simulink model "PowerSplitDriveUnit_harness_model"  (R2022a)
settings: Solver=daessc  StartTime=0.0  StopTime=t_end  RelTol=1e-3  AbsTol=1e-3
PreLoadFcn:
  | PowerSplitDriveUnit_harness_setup
libraries: fl_lib x7, nesl_utility x6, sdl_lib x1
settings Model: Creator=isaacito  LastModifiedBy=isaacito
settings SolverCC: AutoScaleAbsTol=off  AlgebraicLoopSolver=TrustRegion
settings DataIOCC: DSMLogging=off  InspectSignalLogs=on
settings DebuggingCC: UnconnectedInputMsg=warning  UnconnectedOutputMsg=warning  UnconnectedLineMsg=warning  SFMachineParentedDataDiag=warning
settings RTWCC: DLArmComputeVersion=19.05
settings SimscapeCC: SimscapeLogType=all  SimscapeLogSimulationStatistics=on  SimscapeLogLimitData=off

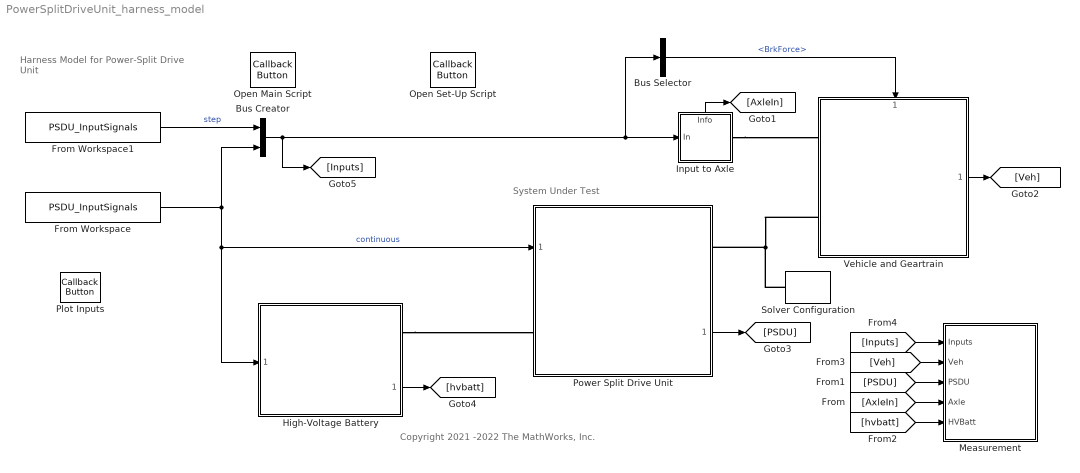
== system PowerSplitDriveUnit_harness_model ==
  note: System Under Test
  note: Copyright 2021 -2022 The MathWorks, Inc.
  note: Harness Model for
      | Power-Split Drive Unit
  Bus Creator : BusCreator  Inputs=2
  Bus Selector : BusSelector  OutputSignals=continuous.BrkForce
  From Workspace : FromWorkspace  VariableName=PSDU_InputSignals  OutDataTypeStr=Bus: PSDU_InputBus  OutputAfterFinalValue=Holding final value
      settings: AttributesFormatString=|
      | %<OutDataTypeStr>
      | Interpolate: %<Interpolate>
  From Workspace1 : FromWorkspace  VariableName=PSDU_InputSignals  OutDataTypeStr=Bus: PSDU_InputBus  Interpolate=off  OutputAfterFinalValue=Holding final value
      settings: AttributesFormatString=|
      | %<OutDataTypeStr>
      | Interpolate: %<Interpolate>
  High-Voltage Battery : Subsystem  ReferencedSubsystem=BatteryForTest2_refsub
      settings: PortSchema="{\"entries\":[{\"content\":{\"sides\":[{\"content\":{\"connectorIds\":[\"In1\"]},\"type\":\"ConnectorPlacement.EquallySpacedRectSide\",\"uuid\":\"6ec42dc2-af13-403d-bb44-bbfe17049ebb\"},{\"content\":{\"connectorIds\":[\"RConn1\",\"Out1\"],\"side\":\"RIGHT\"},\"type\":\"ConnectorPlacement.EquallySpacedRectSide\",\"uuid\":\"18b43a22-b216-415c-b9ff-5dd426481655\"},{\"content\":{\"connectorIds\":[],\"side\":\"TOP\"},\"type\":\"ConnectorPlacement.EquallySpacedRectSide\",\"uuid\":\"9ddf6635-2c27-427a-8c83-df626a0e9ed3\"},{\"content\":{\"connectorIds\":[],\"side\":\"HIDDEN\"},\"type\":\"ConnectorPlacement.EquallySpacedRectSide\",\"uuid\":\"332981be-c8a8-46f3-86be-153015cc7779\"}]},\"type\":\"ConnectorPlacement.EquallySpacedConnector\",\"uuid\":\"0a64d723-305c-452f-a915-e14881ea19f7\"}],\"packageUris\":[\"http://schema.mathworks.com/mf0/Connector/R2020b\"],\"version\":\"1.0\"}"
  Input to Axle : Subsystem
      settings: PortSchema="{\"entries\":[{\"content\":{\"sides\":[{\"content\":{\"connectorIds\":[\"In1\"]},\"type\":\"ConnectorPlacement.EquallySpacedRectSide\",\"uuid\":\"17ecda4f-ad99-4587-a38d-a324d7486455\"},{\"content\":{\"connectorIds\":[\"RConn1\"],\"side\":\"RIGHT\"},\"type\":\"ConnectorPlacement.EquallySpacedRectSide\",\"uuid\":\"02def29b-e53d-45c2-af98-8005350a1631\"},{\"content\":{\"connectorIds\":[\"Out1\"],\"side\":\"TOP\"},\"type\":\"ConnectorPlacement.EquallySpacedRectSide\",\"uuid\":\"2d06855e-5bd1-4c4c-a72f-3146430204d1\"}]},\"type\":\"ConnectorPlacement.EquallySpacedConnector\",\"uuid\":\"a8d07ca5-35bb-4517-a87a-8359777d2cb9\"}],\"packageUris\":[\"http://schema.mathworks.com/mf0/Connector/R2020b\"],\"version\":\"1.0\"}"
  Measurement : Subsystem
  Open Main Script : CallbackButton  ButtonText=Open
      settings: ClickFcn=edit PowerSplitDriveUnit_main_script
  Open Set-Up Script : CallbackButton  ButtonText=Open
      settings: ClickFcn=edit PowerSplitDriveUnit_harness_setup.m
  Plot Inputs : CallbackButton  ButtonText=Plot
      settings: ClickFcn="PowerSplitDriveUnit_plot_inputs(\"PSDU_InputSignals\")"
  Power Split Drive Unit : Subsystem  ReferencedSubsystem=PowerSplitDriveUnitBasic_refsub
      settings: PortSchema="{\"entries\":[{\"content\":{\"sides\":[{\"content\":{\"connectorIds\":[\"In1\",\"LConn1\"]},\"type\":\"ConnectorPlacement.EquallySpacedRectSide\",\"uuid\":\"ac3719a4-f5ca-49c1-b88d-60ddfcbc9c3c\"},{\"content\":{\"connectorIds\":[\"RConn1\",\"Out1\"],\"side\":\"RIGHT\"},\"type\":\"ConnectorPlacement.EquallySpacedRectSide\",\"uuid\":\"02c1cdca-c4bc-4e36-8da7-b9fd13165580\"},{\"content\":{\"connectorIds\":[],\"side\":\"TOP\"},\"type\":\"ConnectorPlacement.EquallySpacedRectSide\",\"uuid\":\"9a293679-982e-42e0-b445-a53b2f9deeb2\"},{\"content\":{\"connectorIds\":[],\"side\":\"HIDDEN\"},\"type\":\"ConnectorPlacement.EquallySpacedRectSide\",\"uuid\":\"92624000-5028-4c46-b75d-fdf82f03c691\"}]},\"type\":\"ConnectorPlacement.EquallySpacedConnector\",\"uuid\":\"49b414d9-6436-4fd3-904c-291d56adec0c\"}],\"packageUris\":[\"http://schema.mathworks.com/mf0/Connector/R2020b\"],\"version\":\"1.0\"}"
  Solver Configuration : nesl_utility/Solver Configuration  PhysicalDomain=network_engine_domain  SubClassName=solver  LeftPortType=input  RightPortType=generic  Tones=[]  Harmonics=[]  SimulateNoise=off  Profile=off  UseLocalSampling=off  EnableSwitchedLinearOptims=on  FrequencyDomain=off  UseCCode=off  RelTol=0.001  AbsTol=1e-06  MinStep=1e-09  ToWorkspace=off  RevertToSquareIcSolve=off  NumHomotopyIterations=100  PhasorMode=off  PhasorModeNumHarmonics=1  IndexReductionMethod=DerivativeReplacement  DoDC=off  ResidualTolerance=1e-09  UseLocalSolver=off  LocalSolverChoice=NE_BACKWARD_EULER_ADVANCER  LocalSolverSampleTime=0.001  DoFixedCost=off  MaxNonlinIter=3  MaxModeIter=2  ComputeImpulses=off  ImpulseIterations=2  LinearAlgebra=auto  LinearAlgebraNumThread=0  EquationFormulation=NE_TIME_EF  DelaysMemoryBudget=1024  AutomaticFiltering=on  FilteringTimeConstant=0.001  PartitionStorageMethod=AS_NEEDED  PartitionMemoryBudget=1024  PartitionMethod=ROBUST
      settings: AttributesFormatString=Local sover: %<UseLocalSolver>  SourceProductBaseCode=SS,PW,VE
  Vehicle and Geartrain : Subsystem  ReferencedSubsystem=VehicleForTest2_refsub
      settings: PortSchema="{\"entries\":[{\"content\":{\"sides\":[{\"content\":{\"connectorIds\":[\"LConn1\",\"LConn2\"]},\"type\":\"ConnectorPlacement.EquallySpacedRectSide\",\"uuid\":\"bb254eee-566f-4c5c-84a7-fb9c4454ad79\"},{\"content\":{\"connectorIds\":[\"Out1\"],\"side\":\"RIGHT\"},\"type\":\"ConnectorPlacement.EquallySpacedRectSide\",\"uuid\":\"f45d8a5c-78f6-4e95-96b7-f45a591913f3\"},{\"content\":{\"connectorIds\":[\"In1\"],\"side\":\"TOP\"},\"type\":\"ConnectorPlacement.EquallySpacedRectSide\",\"uuid\":\"8c3548cd-f99e-45ea-94fd-4a0eb1c6e5ba\"}]},\"type\":\"ConnectorPlacement.EquallySpacedConnector\",\"uuid\":\"bf3d7206-a534-47dd-b57a-354e2e072540\"}],\"packageUris\":[\"http://schema.mathworks.com/mf0/Connector/R2020b\"],\"version\":\"1.0\"}"
  wires:
  Power Split Drive Unit/1 -> [PSDU]
  High-Voltage Battery/1 -> [hvbatt]
  From Workspace/1 -> High-Voltage Battery/1, Power Split Drive Unit/1, Bus Creator/2  "continuous"
  From Workspace1/1 -> Bus Creator/1  "step"
  Vehicle and Geartrain/1 -> [Veh]
  [Veh] -> Measurement/2(Veh)
  [hvbatt] -> Measurement/5(HVBatt)
  [PSDU] -> Measurement/3(PSDU)
  [AxleIn] -> Measurement/4(Axle)
  [Inputs] -> Measurement/1(Inputs)
  Bus Creator/1 -> [Inputs], Bus Selector/1, Input to Axle/1(In)
  Input to Axle/1(Info) -> [AxleIn]
  Bus Selector/1 -> Vehicle and Geartrain/1  "<BrkForce>"
  connections:
  Vehicle and Geartrain/LConn2 -- Solver Configuration/RConn1 -- Power Split Drive Unit/RConn1
  Input to Axle/RConn1 -- Vehicle and Geartrain/LConn1
  High-Voltage Battery/RConn1 -- Power Split Drive Unit/LConn1

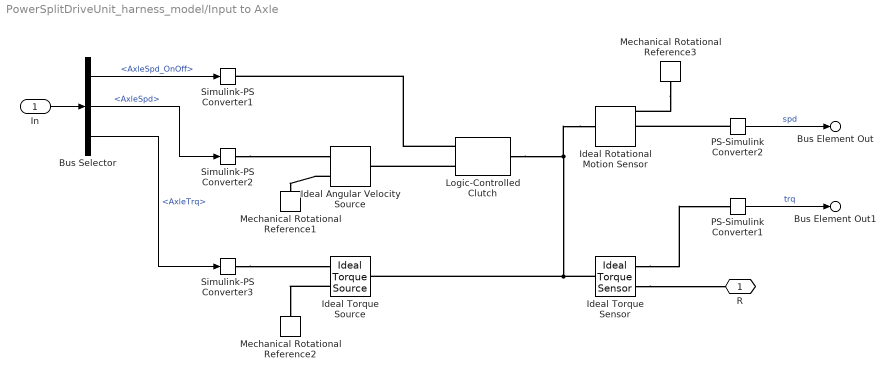
== system PowerSplitDriveUnit_harness_model/Input to Axle ==
  In : Inport
      settings: AttributesFormatString=%<Unit>
  Bus Selector : BusSelector  OutputSignals=step.AxleSpd_OnOff,continuous.AxleSpd,continuous.AxleTrq
  Ideal Angular Velocity Source : fl_lib/Mechanical/Mechanical Sources/Ideal Angular Velocity Source
      settings: SourceProductBaseCode=PW,SS,VE
  Ideal Rotational Motion Sensor : fl_lib/Mechanical/Mechanical Sensors/Ideal Rotational Motion Sensor  wrap_angle=simscape.enum.onoff.off  offset=0 rad
      settings: SourceProductBaseCode=PW,SS,VE
  Ideal Torque Sensor : fl_lib/Mechanical/Mechanical Sensors/Ideal Torque Sensor
      settings: SourceProductBaseCode=PW,SS,VE
  Ideal Torque Source : fl_lib/Mechanical/Mechanical Sources/Ideal Torque Source
      settings: SourceProductBaseCode=PW,SS,VE
  Logic-Controlled Clutch : sdl_lib/Clutches/Logic-Controlled Clutch  transition_model=sdl.enum.transitionModel.instant  transition_time_constant=0.1 s  t_friction=10000 N*m  t_locked=10000 N*m  w_tol=0.001 rad/s  initial_state_locked=sdl.enum.initial_lock.unlocked
      settings: AttributesFormatString=%<initial_state_locked>  SourceProductBaseCode=LD  InternalSimscapePortConfiguration="{\"Bottom\":[],\"Left\":[{\"id\":\"E\",\"label\":\"E\",\"type\":\"input\"},{\"id\":\"B\",\"label\":\"B\",\"type\":\"foundation.mechanical.rotational.rotational\"}],\"Right\":[{\"id\":\"F\",\"label\":\"F\",\"type\":\"foundation.mechanical.rotational.rotational\"}],\"Top\":[]}"
  Mechanical Rotational Reference1 : fl_lib/Mechanical/Rotational Elements/Mechanical Rotational Reference
      settings: SourceProductBaseCode=PW,SS,VE
  Mechanical Rotational Reference2 : fl_lib/Mechanical/Rotational Elements/Mechanical Rotational Reference
      settings: SourceProductBaseCode=PW,SS,VE
  Mechanical Rotational Reference3 : fl_lib/Mechanical/Rotational Elements/Mechanical Rotational Reference
      settings: SourceProductBaseCode=PW,SS,VE
  PS-Simulink Converter1 : nesl_utility/PS-Simulink Converter  PhysicalDomain=network_engine_domain  SubClassName=ps_output  LeftPortType=input  RightPortType=output  PseudoPeriodic=off  Frequencies=[]  VectorFormat=1-D array  Unit=N*m  AffineConversion=off
      settings: SourceProductBaseCode=SS,PW,VE
  PS-Simulink Converter2 : nesl_utility/PS-Simulink Converter  PhysicalDomain=network_engine_domain  SubClassName=ps_output  LeftPortType=input  RightPortType=output  PseudoPeriodic=off  Frequencies=[]  VectorFormat=1-D array  Unit=rpm  AffineConversion=off
      settings: SourceProductBaseCode=SS,PW,VE
  Simulink-PS Converter1 : nesl_utility/Simulink-PS Converter  PhysicalDomain=network_engine_domain  SubClassName=ps_input  LeftPortType=input  RightPortType=output  PseudoPeriodic=off  Frequencies=[]  NoiseDistribution=none  NoiseParameters=[]  Unit=1  AffineConversion=off  FilteringAndDerivatives=provide  SimscapeFilterOrder=1  InputFilterTimeConstant=0.001  UdotUserProvided=0
      settings: SourceProductBaseCode=SS,PW,VE
  Simulink-PS Converter2 : nesl_utility/Simulink-PS Converter  PhysicalDomain=network_engine_domain  SubClassName=ps_input  LeftPortType=input  RightPortType=output  PseudoPeriodic=off  Frequencies=[]  NoiseDistribution=none  NoiseParameters=[]  Unit=rpm  AffineConversion=off  FilteringAndDerivatives=filter  SimscapeFilterOrder=1  InputFilterTimeConstant=0.001  UdotUserProvided=0
      settings: SourceProductBaseCode=SS,PW,VE
  Simulink-PS Converter3 : nesl_utility/Simulink-PS Converter  PhysicalDomain=network_engine_domain  SubClassName=ps_input  LeftPortType=input  RightPortType=output  PseudoPeriodic=off  Frequencies=[]  NoiseDistribution=none  NoiseParameters=[]  Unit=N*m  AffineConversion=off  FilteringAndDerivatives=filter  SimscapeFilterOrder=1  InputFilterTimeConstant=0.001  UdotUserProvided=0
      settings: SourceProductBaseCode=SS,PW,VE
  R : PMIOPort  Side=Right
  Bus Element Out : Outport  PortName=Info  Element=spd
  Bus Element Out1 : Outport  PortName=Info  Element=trq
  wires:
  PS-Simulink Converter2/1 -> Bus Element Out/1  "spd"
  PS-Simulink Converter1/1 -> Bus Element Out1/1  "trq"
  In/1 -> Bus Selector/1
  Bus Selector/1 -> Simulink-PS Converter1/1  "<AxleSpd_OnOff>"
  Bus Selector/2 -> Simulink-PS Converter2/1  "<AxleSpd>"
  Bus Selector/3 -> Simulink-PS Converter3/1  "<AxleTrq>"
  connections:
  Ideal Torque Sensor/RConn2 -- PS-Simulink Converter1/LConn1
  Mechanical Rotational Reference3/LConn1 -- Ideal Rotational Motion Sensor/RConn1
  PS-Simulink Converter2/LConn1 -- Ideal Rotational Motion Sensor/RConn2
  Ideal Rotational Motion Sensor/LConn1 -- Logic-Controlled Clutch/RConn1 -- Ideal Torque Source/LConn1 -- Ideal Torque Sensor/LConn1
  Simulink-PS Converter3/RConn1 -- Ideal Torque Source/RConn1
  Simulink-PS Converter2/RConn1 -- Ideal Angular Velocity Source/RConn1
  Ideal Angular Velocity Source/RConn2 -- Mechanical Rotational Reference1/LConn1
  Logic-Controlled Clutch/LConn2 -- Ideal Angular Velocity Source/LConn1
  Ideal Torque Sensor/RConn1 -- R/RConn1
  Ideal Torque Source/RConn2 -- Mechanical Rotational Reference2/LConn1
  Logic-Controlled Clutch/LConn1 -- Simulink-PS Converter1/RConn1

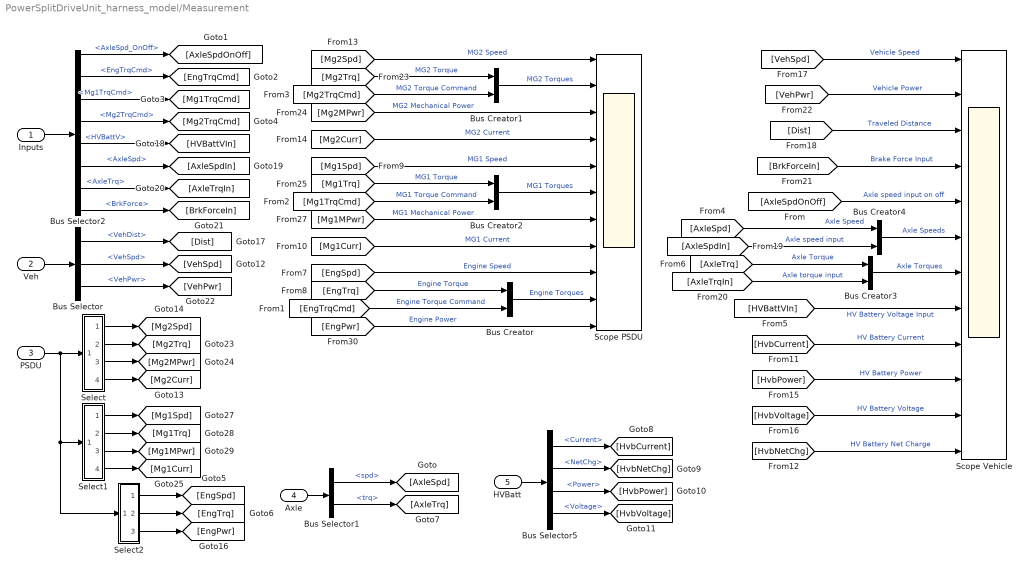
== system PowerSplitDriveUnit_harness_model/Measurement ==
  Inputs : Inport
  Veh : Inport  Port=2
  PSDU : Inport  Port=3
  Axle : Inport  Port=4
  HVBatt : Inport  Port=5
  Bus Creator{,1..4} (5 alike) : BusCreator  Inputs=2
  Bus Selector : BusSelector  OutputSignals=VehDist,VehSpd,VehPwr
  Bus Selector1 : BusSelector  OutputSignals=spd,trq
  Bus Selector2 : BusSelector  OutputSignals=step.AxleSpd_OnOff,continuous.EngTrqCmd,continuous.Mg1TrqCmd,continuous.Mg2TrqCmd,continuous.HVBattV,continuous.AxleSpd,continuous.AxleTrq,continuous.BrkForce
  Bus Selector5 : BusSelector  OutputSignals=Current,NetChg,Power,Voltage
  Scope PSDU : Scope  NumInputPorts=11
  Scope Vehicle : Scope  NumInputPorts=12
  Select : Subsystem
  Select1 : Subsystem
  Select2 : Subsystem
  wires:
  Veh/1 -> Bus Selector/1
  [HvbVoltage] -> Scope Vehicle/11  "HV Battery Voltage"
  [HvbNetChg] -> Scope Vehicle/12  "HV Battery Net Charge"
  [HvbCurrent] -> Scope Vehicle/9  "HV Battery Current"
  [HvbPower] -> Scope Vehicle/10  "HV Battery Power"
  Bus Selector5/1 -> [HvbCurrent]  "<Current>"
  HVBatt/1 -> Bus Selector5/1
  Bus Selector5/3 -> [HvbPower]  "<Power>"
  Bus Selector5/2 -> [HvbNetChg]  "<NetChg>"
  Bus Selector5/4 -> [HvbVoltage]  "<Voltage>"
  Select/4(Mg2Curr) -> [Mg2Curr]
  Select2/2(EngTrq) -> [EngTrq]
  Select2/1(EngSpd) -> [EngSpd]
  Select/1(Mg2Spd) -> [Mg2Spd]
  Axle/1 -> Bus Selector1/1
  Bus Selector1/1 -> [AxleSpd]  "<spd>"
  Bus Selector1/2 -> [AxleTrq]  "<trq>"
  Inputs/1 -> Bus Selector2/1
  Bus Selector2/1 -> [AxleSpdOnOff]  "<AxleSpd_OnOff>"
  Bus Selector2/2 -> [EngTrqCmd]  "<EngTrqCmd>"
  Bus Selector2/3 -> [Mg1TrqCmd]  "<Mg1TrqCmd>"
  Bus Selector2/4 -> [Mg2TrqCmd]  "<Mg2TrqCmd>"
  Bus Selector2/5 -> [HVBattVIn]  "<HVBattV>"
  Bus Selector2/6 -> [AxleSpdIn]  "<AxleSpd>"
  Bus Selector2/7 -> [AxleTrqIn]  "<AxleTrq>"
  Bus Selector2/8 -> [BrkForceIn]  "<BrkForce>"
  [VehSpd] -> Scope Vehicle/1  "Vehicle Speed"
  [Dist] -> Scope Vehicle/3  "Traveled Distance"
  [EngTrq] -> Bus Creator/1  "Engine Torque"
  [EngTrqCmd] -> Bus Creator/2  "Engine Torque Command"
  [HVBattVIn] -> Scope Vehicle/8  "HV Battery Voltage Input"
  [AxleSpdOnOff] -> Scope Vehicle/5  "Axle speed input on off"
  [BrkForceIn] -> Scope Vehicle/4  "Brake Force Input"
  Bus Selector/1 -> [Dist]  "<VehDist>"
  Bus Selector/2 -> [VehSpd]  "<VehSpd>"
  Bus Selector/3 -> [VehPwr]  "<VehPwr>"
  [VehPwr] -> Scope Vehicle/2  "Vehicle Power"
  Select/2(Mg2Trq) -> [Mg2Trq]
  Select/3(Mg2MechPwr) -> [Mg2MPwr]
  [Mg2Trq] -> Bus Creator1/1  "MG2 Torque"
  [Mg2TrqCmd] -> Bus Creator1/2  "MG2 Torque Command"
  [Mg2Spd] -> Scope PSDU/1  "MG2 Speed"
  Bus Creator1/1 -> Scope PSDU/2  "MG2 Torques"
  [Mg2MPwr] -> Scope PSDU/3  "MG2 Mechanical Power"
  Select1/1(Mg1Spd) -> [Mg1Spd]
  Select1/2(Mg1Trq) -> [Mg1Trq]
  Select1/3(Mg1MechPwr) -> [Mg1MPwr]
  Select1/4(Mg1Curr) -> [Mg1Curr]
  [Mg1Trq] -> Bus Creator2/1  "MG1 Torque"
  [Mg1TrqCmd] -> Bus Creator2/2  "MG1 Torque Command"
  PSDU/1 -> Select2/1(PSDU), Select1/1(PSDU), Select/1(PSDU)
  Select2/3(EngPwr) -> [EngPwr]
  [AxleTrq] -> Bus Creator3/1  "Axle Torque"
  [AxleTrqIn] -> Bus Creator3/2  "Axle torque input"
  Bus Creator3/1 -> Scope Vehicle/7  "Axle Torques"
  [AxleSpdIn] -> Bus Creator4/2  "Axle speed input"
  [AxleSpd] -> Bus Creator4/1  "Axle Speed"
  Bus Creator4/1 -> Scope Vehicle/6  "Axle Speeds"
  [Mg2Curr] -> Scope PSDU/4  "MG2 Current"
  [Mg1Spd] -> Scope PSDU/5  "MG1 Speed"
  Bus Creator2/1 -> Scope PSDU/6  "MG1 Torques"
  [Mg1MPwr] -> Scope PSDU/7  "MG1 Mechanical Power"
  [Mg1Curr] -> Scope PSDU/8  "MG1 Current"
  [EngSpd] -> Scope PSDU/9  "Engine Speed"
  Bus Creator/1 -> Scope PSDU/10  "Engine Torques"
  [EngPwr] -> Scope PSDU/11  "Engine Power"

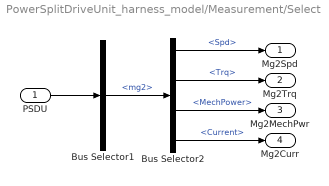
== system PowerSplitDriveUnit_harness_model/Measurement/Select ==
  PSDU : Inport
  Bus Selector1 : BusSelector  OutputSignals=mg2
  Bus Selector2 : BusSelector  OutputSignals=Spd,Trq,MechPower,Current
  Mg2Spd : Outport
  Mg2Trq : Outport  Port=2
  Mg2MechPwr : Outport  Port=3
  Mg2Curr : Outport  Port=4
  wires:
  PSDU/1 -> Bus Selector1/1
  Bus Selector1/1 -> Bus Selector2/1  "<mg2>"
  Bus Selector2/1 -> Mg2Spd/1  "<Spd>"
  Bus Selector2/4 -> Mg2Curr/1  "<Current>"
  Bus Selector2/2 -> Mg2Trq/1  "<Trq>"
  Bus Selector2/3 -> Mg2MechPwr/1  "<MechPower>"

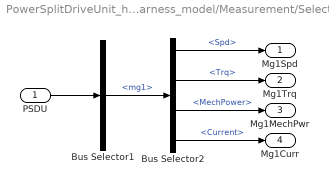
== system PowerSplitDriveUnit_harness_model/Measurement/Select1 ==
  PSDU : Inport
  Bus Selector1 : BusSelector  OutputSignals=mg1
  Bus Selector2 : BusSelector  OutputSignals=Spd,Trq,MechPower,Current
  Mg1Spd : Outport
  Mg1Trq : Outport  Port=2
  Mg1MechPwr : Outport  Port=3
  Mg1Curr : Outport  Port=4
  wires:
  PSDU/1 -> Bus Selector1/1
  Bus Selector1/1 -> Bus Selector2/1  "<mg1>"
  Bus Selector2/1 -> Mg1Spd/1  "<Spd>"
  Bus Selector2/4 -> Mg1Curr/1  "<Current>"
  Bus Selector2/2 -> Mg1Trq/1  "<Trq>"
  Bus Selector2/3 -> Mg1MechPwr/1  "<MechPower>"

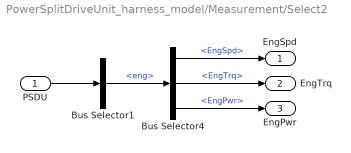
== system PowerSplitDriveUnit_harness_model/Measurement/Select2 ==
  PSDU : Inport
  Bus Selector1 : BusSelector  OutputSignals=eng
  Bus Selector4 : BusSelector  OutputSignals=EngSpd,EngTrq,EngPwr
  EngSpd : Outport
  EngTrq : Outport  Port=2
  EngPwr : Outport  Port=3
  wires:
  PSDU/1 -> Bus Selector1/1
  Bus Selector1/1 -> Bus Selector4/1  "<eng>"
  Bus Selector4/1 -> EngSpd/1  "<EngSpd>"
  Bus Selector4/2 -> EngTrq/1  "<EngTrq>"
  Bus Selector4/3 -> EngPwr/1  "<EngPwr>"
